simulink model "cascade"  (R2016a)
settings: Solver=VariableStepAuto  StartTime=0.0  StopTime=5  RelTol=1e-3
libraries: powerlib x14
settings Model: Creator=Diksha  LastModifiedBy=Admin

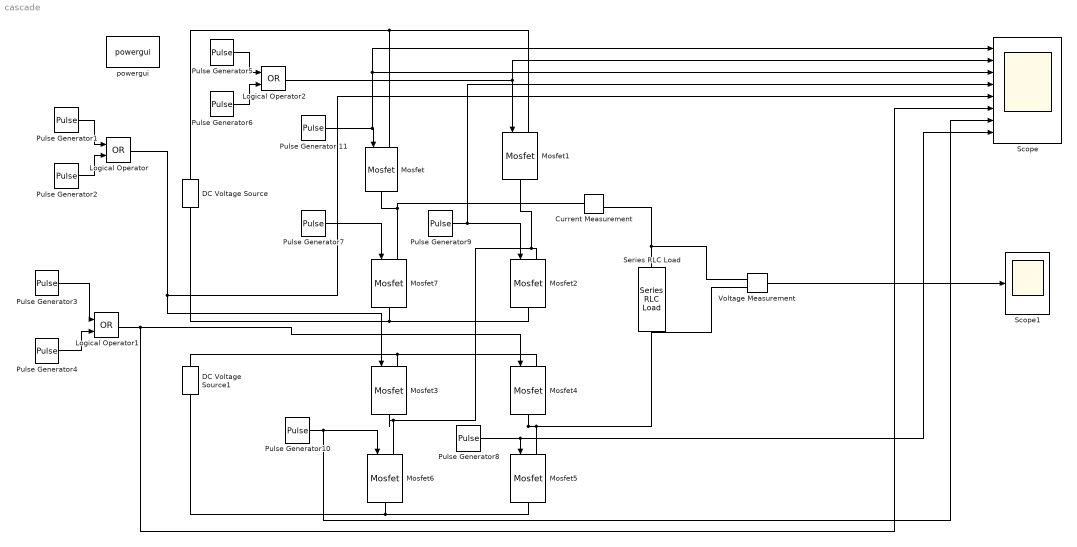
== system cascade ==
  Current Measurement : powerlib/Measurements/Current Measurement  PhasorSimulation=off  OutputType=Complex  PSBequivalent=0
  DC Voltage Source : powerlib/Electrical Sources/DC Voltage Source  Amplitude=100  Measurements=None
  DC Voltage Source1 : powerlib/Electrical Sources/DC Voltage Source  Amplitude=100  Measurements=None
  Logical Operator : Logic  Operator=OR  AllPortsSameDT=off  OutDataTypeStr=boolean
  Logical Operator1 : Logic  Operator=OR  AllPortsSameDT=off  OutDataTypeStr=boolean
  Logical Operator2 : Logic  Operator=OR  AllPortsSameDT=off  OutDataTypeStr=boolean
  Mosfet{,1..7} (8 alike) : powerlib/Power Electronics/Mosfet  Ron=0.1  Lon=0  Rd=0.01  Vfd=0  IC=0  Rs=1e5  Cs=inf  Measurements=off
  Pulse Generator 11 : DiscretePulseGenerator  PulseType=Time based  Period=0.02  PulseWidth=(5/8)*100  PhaseDelay=(0.02/8)*0
  Pulse Generator1 : DiscretePulseGenerator  PulseType=Time based  Period=0.02  PulseWidth=(6/8)*100  PhaseDelay=(0.02/8)*0
  Pulse Generator10 : DiscretePulseGenerator  PulseType=Time based  Period=0.02  PulseWidth=(1/8)*100  PhaseDelay=(0.02/8)*6
  Pulse Generator2 : DiscretePulseGenerator  PulseType=Time based  Period=0.02  PulseWidth=(1/8)*100  PhaseDelay=(0.02/8)*7
  Pulse Generator3 : DiscretePulseGenerator  PulseType=Time based  Period=0.02  PulseWidth=(2/8)*100  PhaseDelay=(0.02/8)*0
  Pulse Generator4 : DiscretePulseGenerator  PulseType=Time based  Period=0.02  PulseWidth=(5/8)*100  PhaseDelay=(0.02/8)*3
  Pulse Generator5 : DiscretePulseGenerator  PulseType=Time based  Period=0.02  PulseWidth=(1/8)*100  PhaseDelay=(0.02/8)*0
  Pulse Generator6 : DiscretePulseGenerator  PulseType=Time based  Period=0.02  PulseWidth=(4/8)*100  PhaseDelay=(0.02/8)*4
  Pulse Generator7 : DiscretePulseGenerator  PulseType=Time based  Period=0.02  PulseWidth=(3/8)*100  PhaseDelay=(0.02/8)*5
  Pulse Generator8 : DiscretePulseGenerator  PulseType=Time based  Period=0.02  PulseWidth=(1/8)*100  PhaseDelay=(0.02/8)*2
  Pulse Generator9 : DiscretePulseGenerator  PulseType=Time based  Period=0.02  PulseWidth=(3/8)*100  PhaseDelay=(0.02/8)*1
  Scope : Scope  NumInputPorts=8
  Scope1 : Scope
  Series RLC Load : powerlib/Elements/Series RLC Load  LConnTagsString=a  RConnTagsString=__new0  NominalVoltage=1000  NominalFrequency=60  ActivePower=10e3  InductivePower=0  CapacitivePower=0  Setx0=off  InitialVoltage=0  SetiL0=off  InitialCurrent=0  Measurements=None  LoadType=constant Z
  Voltage Measurement : powerlib/Measurements/Voltage Measurement  PhasorSimulation=off  OutputType=Complex  PSBequivalent=0
  powergui : powerlib/powergui  Priority=1  SimulationMode=Continuous  SolverType=Tustin/Backward Euler (TBE)  SampleTime=50e-6  frequency=60  SPID=off  DisableSnubberDevices=off  DisableRonSwitches=off  DisableVfSwitches=off  SwTol=0  DisplayEquations=off  Interpol=off  ExternalGateDelay=off  methode=off  Ts=10  FunctionMessages=off  echomessages=off  HookPort=off  EnableUseOfTLC=off  x0status=blocks  frequencyindice=0  Pbase=100e6  ErrMax=1e-4  Iterations=50  UnitsV=kV  UnitsW=MW  buscounter=0  RestoreLinks=warning  ResistiveCurrentMeasurement=off  Frange=[0:2:500]  Ylog=off  Xlog=on  ShowGrid=off  save=off  variable=ZData  structure=0  ZoomFFT=off  StartTime=0.0  cycles=1  DisplayStyle=1  fundamental=60  FreqAxis=off  MaxFrequency=1000  frequencyindicesteady=1  RmsSteady=1  display=off
  wires:
  Pulse Generator1/1 -> Logical Operator/1
  Pulse Generator2/1 -> Logical Operator/2
  Pulse Generator3/1 -> Logical Operator1/1
  Pulse Generator4/1 -> Logical Operator1/2
  Pulse Generator5/1 -> Logical Operator2/1
  Pulse Generator6/1 -> Logical Operator2/2
  Pulse Generator 11/1 -> Scope/3, Scope/1, Mosfet/1
  Pulse Generator8/1 -> Scope/8, Mosfet5/1
  Pulse Generator10/1 -> Mosfet6/1, Scope/7
  Voltage Measurement/1 -> Scope1/1
  Pulse Generator7/1 -> Mosfet7/1
  Logical Operator/1 -> Scope/5, Mosfet3/1
  Logical Operator1/1 -> Scope/6, Mosfet4/1
  Logical Operator2/1 -> Mosfet1/1, Scope/2
  Pulse Generator9/1 -> Scope/4, Mosfet2/1
  connections:
  DC Voltage Source/RConn1 -- Mosfet/LConn1 -- Mosfet1/LConn1
  DC Voltage Source/LConn1 -- Mosfet7/RConn1 -- Mosfet2/RConn1
  DC Voltage Source1/RConn1 -- Mosfet3/LConn1 -- Mosfet4/LConn1
  DC Voltage Source1/LConn1 -- Mosfet6/RConn1 -- Mosfet5/RConn1
  Mosfet3/RConn1 -- Mosfet2/LConn1 -- Mosfet1/RConn1 -- Mosfet6/LConn1
  Current Measurement/LConn1 -- Mosfet/RConn1 -- Mosfet7/LConn1
  Mosfet4/RConn1 -- Voltage Measurement/LConn2 -- Series RLC Load/RConn1 -- Mosfet5/LConn1
  Current Measurement/RConn1 -- Voltage Measurement/LConn1 -- Series RLC Load/LConn1
